simulink model "Manifold_and_Nozzle_Model"  (R2023b)
settings: Solver=VariableStepAuto  StartTime=0.0  StopTime=1000  FixedStep=0.01  RelTol=1e-3
undefined symbols (not defined in the file): P_amb, P_init, T_amb, T_init
libraries: fl_lib x9, nesl_utility x4
(part 2 of 2)

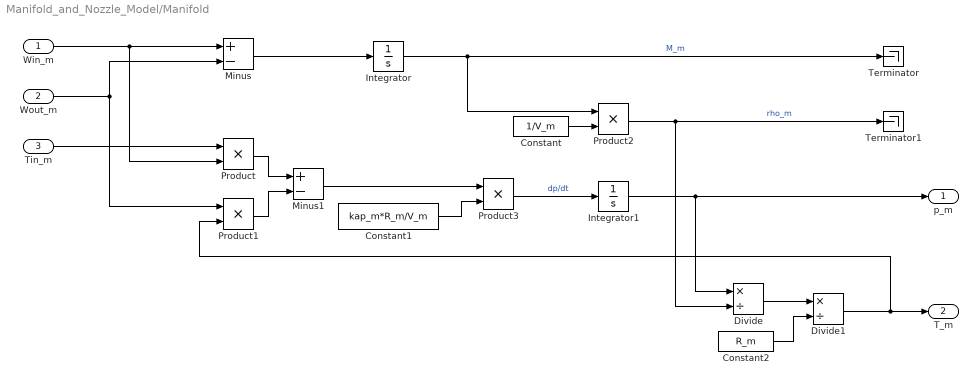
== system Manifold_and_Nozzle_Model/Manifold ==
  Win_m : Inport
  Wout_m : Inport  Port=2
  Tin_m : Inport  Port=3
  Constant : Constant  Value=1/V_m
  Constant1 : Constant  Value=kap_m*R_m/V_m
  Constant2 : Constant  Value=R_m
  Divide : Product  Inputs=*/
  Divide1 : Product  Inputs=*/
  Integrator : Integrator  InitialCondition=P_init*V_m/(R_m*T_init)
  Integrator1 : Integrator  InitialCondition=P_init
  Minus : Sum  Inputs=+-
  Minus1 : Sum  Inputs=+-
  Product{,1..3} (4 alike) : Product
  Terminator : Terminator
  Terminator1 : Terminator
  p_m : Outport
  T_m : Outport  Port=2
  wires:
  Win_m/1 -> Minus/1, Product/2
  Wout_m/1 -> Product1/1, Minus/2
  Minus/1 -> Integrator/1
  Integrator/1 -> Product2/1, Terminator/1  "M_m"
  Product2/1 -> Terminator1/1, Divide/2  "rho_m"
  Tin_m/1 -> Product/1
  Product/1 -> Minus1/1
  Product1/1 -> Minus1/2
  Minus1/1 -> Product3/1
  Constant/1 -> Product2/2
  Constant1/1 -> Product3/2
  Integrator1/1 -> p_m/1, Divide/1
  Constant2/1 -> Divide1/2
  Divide1/1 -> Product1/2, T_m/1
  Divide/1 -> Divide1/1
  Product3/1 -> Integrator1/1  "dp/dt"

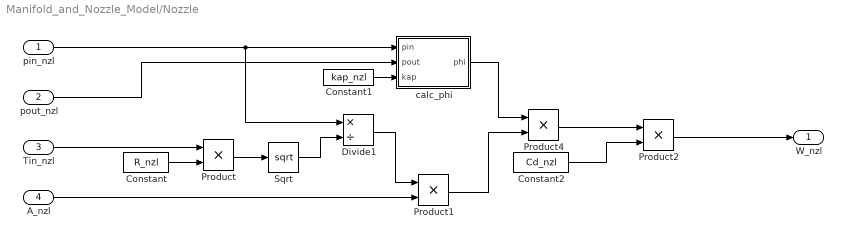
== system Manifold_and_Nozzle_Model/Nozzle ==
  pin_nzl : Inport
  pout_nzl : Inport  Port=2
  Tin_nzl : Inport  Port=3
  A_nzl : Inport  Port=4
  Constant : Constant  Value=R_nzl
  Constant1 : Constant  Value=kap_nzl
  Constant2 : Constant  Value=Cd_nzl
  Divide1 : Product  Inputs=*/
  Product{,1..2,4} (4 alike) : Product
  Sqrt : Sqrt
  calc_phi : MATLAB Function  TreatAsAtomicUnit=on
  W_nzl : Outport
  wires:
  pout_nzl/1 -> calc_phi/2(pout)
  pin_nzl/1 -> calc_phi/1(pin), Divide1/1
  Tin_nzl/1 -> Product/1
  A_nzl/1 -> Product1/2
  Constant/1 -> Product/2
  Product/1 -> Sqrt/1
  Sqrt/1 -> Divide1/2
  Divide1/1 -> Product1/1
  Constant1/1 -> calc_phi/3(kap)
  calc_phi/1(phi) -> Product4/1
  Product1/1 -> Product4/2
  Product4/1 -> Product2/1
  Product2/1 -> W_nzl/1
  Constant2/1 -> Product2/2

== matlab function Manifold_and_Nozzle_Model/Nozzle/calc_phi ==
  data: pin input; phi output; pout input; kap input
function phi = fcn(pin,pout,kap)
    pr = pout/pin;
    p_cr = (2/(kap+1))^(kap/(kap-1))*pin;
    % Judge critical pressure
    if pout < p_cr
        tmp_phi = sqrt(kap*(2/(kap+1))^((kap+1)/(kap-1)));
    else
        tmp_phi = pr^(1/kap)*sqrt(2*kap/(kap-1)*(1-pr^((kap-1)/kap)));
    end
    phi = tmp_phi;
end
